simulink model "QDiff_ASGSM"  (R2024b)
settings: Solver=ode4  StartTime=0.0  StopTime=5  FixedStep=0.004  RelTol=1e-3
undefined symbols (not defined in the file or in its folder): DiscIntNeverNeededParam
libraries: aerolibutil x9, sharedutil x3, matrix_library x2, simulink_extras x1, simulink x1, sharedtransform x1
settings Model: Creator=danyy  LastModifiedBy=danyy

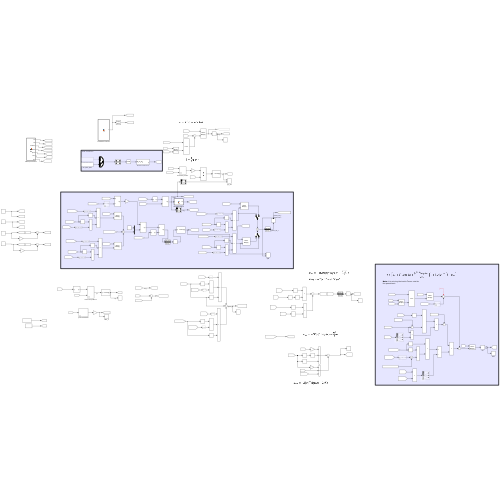
[thumbnail: Simulink's stored preview of the top-level diagram]
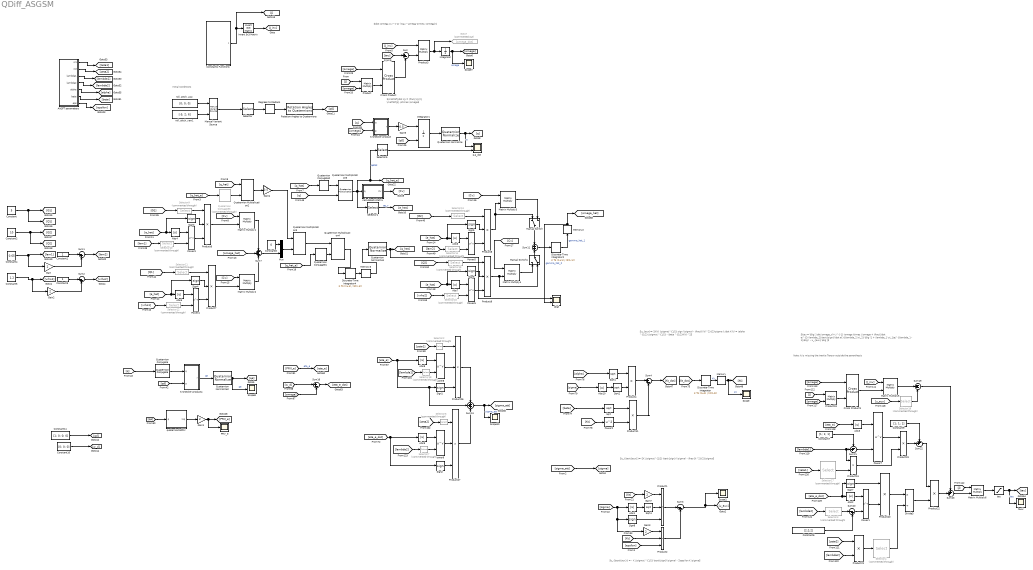
== system QDiff_ASGSM ==
  note: $u_{\text{aux}} = - K |\sigma| ^{1/2} \text{sign}(\sigma) - 2\epsilon K \sigma$
  note: $u_{\text{aux}}=-2K |\sigma|^{1/2} \text{sign} (\sigma) - \frac{K^2}{2}\sigma$
  note: $u_{aux}=-2K(t) |\sigma|^{1/2} sign (\sigma) - \frac{K(t)^2}{2}\sigma \\ \dot K(t) = \alpha ^{1/2} |\sigma| ^{1/2} - \beta ^{1/2}K(t)^2$
  note: $\tau = \Big [ \dot \omega_d + J^{-1} \omega \times J \omega + \frac{|\dot e|^{2-\lambda_2}\text{sign}(\dot e)}{\lambda_2 \xi_2} \Big (1 + \lambda_1 \xi_1|e|^{\lambda_1 - 1}\Big ) - u_{aux} \Big ]$
  note: Note: It is missing the Inertia Tensor outside
      | the parenthesis
  note: $\mathbf{\dot q} = \frac{1}{2} \mathbf{q} \otimes \omega$
  note: $\dot \omega = J^{-1} (\tau - \omega \times J \omega)$
  note: Initial Conditions
  ANSFT parameters : MATLAB Function  TreatAsAtomicUnit=on
  Abs{1..10} (10 alike) : Abs  SaturateOnIntegerOverflow=off
  Constant : Constant  Value=5
  Constant1 : Constant
  Constant10 : Constant  Value=[0; 0; 0]
  Constant11 : Constant  Value=[1; 0; 0; 0]
  Constant2 : Constant  Value=10
  Constant3 : Constant
  Constant4 : Constant  Value=0.65
  Constant5 : Constant  Value=1.2
  Constant6 : Constant  Value=[2;2;2]
  Constant7 : Constant  Value=[1; 1; 1]
  Constant8 : Constant  Value=0
  Constant9 : Constant  Value=[1; 1; 1]
  Constants Functions : MATLAB Function  TreatAsAtomicUnit=on
  Cross Product : matrix_library/Cross Product
  Cross Product1 : matrix_library/Cross Product
  Degrees to Radians : simulink_extras/Transformations/Degrees to Radians
  Discrete-Time Integrator : DiscreteIntegrator  IntegratorMethod=Integration: Trapezoidal  InitialCondition=[0; 0; 0]  SampleTime=0.004  ICPrevOutput=DiscIntNeverNeededParam  ICPrevScaledInput=DiscIntNeverNeededParam
  Discrete-Time Integrator2 : DiscreteIntegrator  IntegratorMethod=Integration: Trapezoidal  InitialCondition=[0; 0; 0]  SampleTime=0.004  ICPrevOutput=DiscIntNeverNeededParam  ICPrevScaledInput=DiscIntNeverNeededParam
  Discrete-Time Integrator4 : DiscreteIntegrator  IntegratorMethod=Integration: Trapezoidal  InitialCondition=[1; 0; 0; 0]  SampleTime=0.004  ICPrevOutput=DiscIntNeverNeededParam  ICPrevScaledInput=DiscIntNeverNeededParam
  Divide3 : Product  Inputs=*/
  Gain{,1..3,7} (5 alike) : Gain  Gain=2
  Gain4 : Gain  Gain=0.5
  Gain5 : Gain  Gain=0.5
  Goto7 : Goto  Commented=on  GotoTag=omega_dot
  Integrator : Integrator  InitialCondition=[0; 0; 0]
  Integrator1 : Integrator  InitialConditionSource=external
  Invert 3x3 Matrix : aerolibutil/Invert  3x3 Matrix
  Kronecker product : Subsystem
      mask Display: image('$imagefile'); % Use "Edit Image" on toolstrip to change.
  Kronecker product4 : Subsystem
  Manual Variant Source : simulink/Signal Routing/Manual Variant Source  NumChoices=2  LabelModeActiveChoice=V_2
  Manual Switch : ManualSwitch
  Manual Switch1 : ManualSwitch  CurrentSetting=0
  Matrix Multiply{1..6} (6 alike) : Product  Multiplication=Matrix(*)
  Memory : Memory  InitialCondition=[0; 0; 0]  InheritSampleTime=on
  Memory2 : Memory  InitialCondition=[0; 0; 0]  InheritSampleTime=on
  Memory3 : Memory  InitialCondition=[1; 0; 0; 0]  InheritSampleTime=on
  Mux : Mux  Inputs=2
  PRV_e : Scope
  Power{1,3..9} (8 alike) : Math  Operator=pow
  Power2 : Math  Operator=square
  Product : Product  Multiplication=Matrix(*)
  Product{1..2,6..9,26..27} (8 alike) : Product  Inputs=3
  Product{4,11,20..24} (7 alike) : Product
  Product19 : Product  Multiplication=Matrix(*)
  Product3 : Product  Multiplication=Matrix(*)
  Quaternion Conjugate : aerolibutil/Quaternion Conjugate
  Quaternion Conjugate1 : aerolibutil/Quaternion Conjugate
  Quaternion Conjugate2 : aerolibutil/Quaternion Conjugate
  Quaternion Conjugate3 : aerolibutil/Quaternion Conjugate  Commented=through
  Quaternion Multiplication{2..5} (4 alike) : aerolibutil/Quaternion Multiplication
  Quaternion Normalize : sharedutil/Quaternion Normalize  aMode=aMode
  Quaternion Normalize1 : sharedutil/Quaternion Normalize  aMode=aMode
  Quaternion Normalize2 : sharedutil/Quaternion Normalize  aMode=aMode
  Rotation Angles to Quaternions : sharedtransform/Rotation Angles to Quaternions  rotationOrder=ZYX  aMode=aMode
  Scope{,1,7..8,10} (5 alike) : Scope
  Selector : Selector  InputPortWidth=3  IndexOptions=Index vector (dialog)  Indices=[3 2 1]  OutputSizes=1
  Selector1 : Selector  InputPortWidth=4  IndexOptions=Index vector (dialog)  Indices=[2:4]  OutputSizes=1
  Selector{2..4,6..7,9..19} (16 alike) : Selector  Commented=through  InputPortWidth=6  IndexOptions=Index vector (dialog)  Indices=[4:6]  OutputSizes=1
  Selector5 : Selector  InputPortWidth=4  IndexOptions=Index vector (dialog)  Indices=[2:4]  OutputSizes=1
  Sign{1..8} (8 alike) : Signum
  Sqrt{,1..2,4} (4 alike) : Sqrt
  Sum : Sum  Inputs=|+-
  Sum1 : Sum  Inputs=|-+
  Sum11 : Sum  Inputs=+|+
  Sum16 : Sum  Inputs=|+-
  Sum19 : Sum  Inputs=-+-
  Sum2 : Sum  Inputs=|-+
  Sum20 : Sum  Inputs=|-+
  Sum21 : Sum  Inputs=-+|
  Sum22 : Sum  Inputs=++|
  Sum23 : Sum  Inputs=++|
  Sum24 : Sum  Inputs=+++
  Sum3 : Sum  Inputs=|--
  Sum4 : Sum  Inputs=|+-
  Sum7 : Sum  Inputs=+++
  calculateCvMatrix : MATLAB Function  TreatAsAtomicUnit=on
  q,q_dot : Scope  NumInputPorts=2
  qhat : Scope  NumInputPorts=2
  quaterniontoPRV : Subsystem
  "roll, pitch, yaw" : Constant  Value=[0; 0; 0]
  "roll, pitch, yaw1" : Constant  Value=[-3; 2; 6]
  tau : Saturate
  tauU : Scope
  wires:
  Memory3/1 -> Quaternion Normalize1/1
  [lam2] -> Selector14/1
  Sign6/1 -> Product9/2
  Selector10/1 -> Power3/2
  [G2] -> Selector13/1
  [q_hat_e] -> Quaternion Conjugate1/1
  Selector13/1 -> Product8/1
  Sign4/1 -> Product7/2
  Product6/1 -> Matrix Multiply1/2
  Selector15/1 -> Product9/1
  [Q1] -> Selector11/1
  Product7/1 -> Matrix Multiply2/2
  [Q2] -> Selector15/1
  [Cv] -> Matrix Multiply2/1
  Abs7/1 -> Power6/1
  [e_hat] -> Sign6/1, Abs7/1
  Quaternion Conjugate3/1 -> Quaternion Multiplication2/2
  Sign5/1 -> Product8/2
  Mux/1 -> Quaternion Multiplication3/2
  Matrix Multiply1/1 -> Sum7/1
  [q_hat] -> Quaternion Multiplication2/1
  Selector12/1 -> Power4/2
  Abs6/1 -> Power5/1
  Quaternion Conjugate1/1 -> Quaternion Multiplication4/2
  Power6/1 -> Product9/3
  Selector9/1 -> Product6/1
  Quaternion Multiplication2/1 -> Gain4/1
  [e_hat] -> Sign3/1, Abs4/1
  Power3/1 -> Product6/3
  Selector14/1 -> Power5/2
  Selector16/1 -> Power6/2
  Memory2/1 -> qhat/2, [omega_hat]  "gamma_hat_2"
  Constant8/1 -> Mux/1
  Quaternion Multiplication4/1 -> Discrete-Time Integrator4/1
  Abs5/1 -> Power4/1
  [Cv] -> Matrix Multiply1/1
  Gain4/1 -> Quaternion Multiplication3/1
  Sum7/1 -> Mux/2
  Power5/1 -> Product8/3
  [vrho2] -> Selector16/1
  Matrix Multiply2/1 -> Sum7/3
  [q_hat_e] -> Quaternion Conjugate3/1
  [e_hat] -> Sign5/1, Abs6/1
  Selector11/1 -> Product7/1
  Quaternion Normalize1/1 -> qhat/1, [q_hat]
  Discrete-Time Integrator2/1 -> Memory2/1  "gamma_hat_1"
  Product9/1 -> Manual Switch1/2, Matrix Multiply4/2
  [vrho1] -> Selector12/1
  [Cv] -> Matrix Multiply3/1
  Power4/1 -> Product7/3
  Matrix Multiply3/1 -> Manual Switch/2
  Matrix Multiply4/1 -> Manual Switch1/1
  Product8/1 -> Manual Switch/1, Matrix Multiply3/2
  [lam1] -> Selector10/1
  Discrete-Time Integrator4/1 -> Memory3/1
  [e_hat] -> Sign4/1, Abs5/1
  [G1] -> Selector9/1
  Abs4/1 -> Power3/1
  Sign3/1 -> Product6/2
  Quaternion Multiplication3/1 -> Quaternion Multiplication4/1
  Sum11/1 -> Discrete-Time Integrator2/1
  [omega_hat] -> Sum7/2
  [Cv] -> Matrix Multiply4/1
  Constant3/1 -> Sum2/1
  Constant/1 -> [G1], [Q1]
  Gain/1 -> Sum1/2
  Constant5/1 -> Gain2/1, [vrho1]
  Constant1/1 -> Sum1/1
  Gain2/1 -> Sum2/2
  Sum2/1 -> [vrho2]
  Constant4/1 -> Gain/1, [lam1]
  Constant2/1 -> [G2], [Q2]
  Sum1/1 -> [lam2]
  [q] -> Quaternion Multiplication5/2
  calculateCvMatrix/1(Cv) -> [Cv]
  [q_hat] -> Quaternion Conjugate2/1
  Quaternion Conjugate2/1 -> Quaternion Multiplication5/1
  Quaternion Multiplication5/1 -> Selector1/1, calculateCvMatrix/1(q), Selector5/1, [q_hat_e]  "qehat"
  Selector1/1 -> [e_hat]  "qe_v"
  Kronecker product4/1(r) -> Quaternion Normalize2/1  "qe"
  [qd] -> Kronecker product4/2(p)
  quaterniontoPRV/1(lnq) -> Gain1/1
  Quaternion Normalize2/1 -> Scope8/1, [qe]  "qe"
  Quaternion Conjugate/1 -> Kronecker product4/1(q)
  [q] -> Quaternion Conjugate/1
  [qe] -> quaterniontoPRV/1(q)
  Gain1/1 -> PRV_e/1, [PRV_e]
  [PRV_e] -> [eta_e]  "eta_e"
  [w_d] -> Sum16/1
  [omega] -> Sum16/2
  Sum16/1 -> [eta_e_dot]
  Product27/1 -> Sum24/3
  Selector18/1 -> Power8/2
  Selector6/1 -> Product27/1
  [eta_e] -> Sum24/2, Sign1/1, Abs8/1
  Selector7/1 -> Power9/2
  Abs8/1 -> Power8/1
  [eta_e_dot] -> Abs9/1, Sign2/1
  [lambda2] -> Selector7/1
  [lambda1] -> Selector18/1
  Product26/1 -> Sum24/1
  [zeta2] -> Selector6/1
  Abs9/1 -> Power9/1
  [zeta1] -> Selector2/1
  Sum24/1 -> Scope10/1, [sigma_att]  "sigma_att"
  Selector2/1 -> Product26/1
  Sign2/1 -> Product27/3
  Power9/1 -> Product27/2
  Sign1/1 -> Product26/3
  Power8/1 -> Product26/2
  Gain3/1 -> Product2/1
  Sum4/1 -> [Kt_dot]
  Sum3/1 -> Scope1/1, [u_aux]
  [Kt_dot] -> Discrete-Time Integrator/1
  [Kt] -> Power2/1
  [beta] -> Sqrt/1
  Product11/1 -> Sum4/2
  Product2/1 -> Sum3/2
  [Kt] -> Gain7/1
  [sigma_att] -> [sigma]
  Sign8/1 -> Product1/3
  Sqrt1/1 -> Product4/1
  [alpha] -> Sqrt1/1
  Power2/1 -> Product11/2
  Memory/1 -> Scope/1, [Kt]  "Kt"
  Gain7/1 -> Product1/1
  [sigma] -> Abs10/1
  [epsilon] -> Product2/3
  Product1/1 -> Sum3/1
  Abs10/1 -> Sqrt2/1
  Product4/1 -> Sum4/1
  Sqrt/1 -> Product11/1
  Sqrt2/1 -> Product4/2
  Discrete-Time Integrator/1 -> Memory/1  "Kt"
  [Kt] -> Product2/2
  Sqrt4/1 -> Product1/2
  [sigma] -> Abs1/1, Gain3/1, Sign8/1
  Abs1/1 -> Sqrt4/1
  Product23/1 -> Sum22/2
  Sum22/1 -> Product22/1
  Product20/1 -> Divide3/1
  ? -> Sum19/1
  Matrix Multiply5/1 -> Sum19/2
  Matrix Multiply6/1 -> tau/1
  [lambda2] -> Selector3/1
  Product21/1 -> Selector4/1
  Sum21/1 -> Power7/2
  [lambda1] -> Product24/1, Sum21/2
  Constant9/1 -> Sum22/1
  [J_inv] -> Matrix Multiply5/1
  [J] -> Product19/1
  [u_aux] -> Selector19/1
  Product19/1 -> Cross Product1/2
  [lambda2] -> Product21/2
  tau/1 -> tauU/1, [tau]  "tau"
  Sum23/1 -> Matrix Multiply6/2
  Constant6/1 -> Sum20/2
  [eta_e_dot] -> Sign7/1, Abs2/1
  Cross Product1/1 -> Matrix Multiply5/2
  Selector19/1 -> Sum19/3
  Selector4/1 -> Divide3/2
  [eta_e] -> Abs3/1
  Sum19/1 -> Sum23/1
  [omega] -> Product19/2
  [zeta2] -> Product21/1
  Abs2/1 -> Power1/1
  Constant7/1 -> Sum21/1
  Power7/1 -> Product23/1
  Selector17/1 -> Product24/2
  [J] -> Matrix Multiply6/1
  [omega] -> Cross Product1/1
  Sum20/1 -> Power1/2
  Sign7/1 -> Product20/1
  Product22/1 -> Sum23/2
  [zeta1] -> Selector17/1
  Product24/1 -> Product23/2
  Selector3/1 -> Sum20/1
  Divide3/1 -> Product22/2
  Power1/1 -> Product20/2
  Abs3/1 -> Power7/1
  Product3/1 -> Goto7/1, Integrator/1
  [q] -> Kronecker product/1(q)
  [omega] -> Cross Product/1
  Sum/1 -> Product3/2
  [omega] -> Kronecker product/2(p)
  [omega] -> Product/2
  Quaternion Normalize/1 -> q,q_dot/1, [q]  "q"
  Product/1 -> Cross Product/2
  Integrator1/1 -> Quaternion Normalize/1
  Cross Product/1 -> Sum/2
  Integrator/1 -> Scope7/1, [omega]  "omega"
  [tau] -> Sum/1
  [q0] -> Integrator1/2
  [J_inv] -> Product3/1
  Gain5/1 -> Integrator1/1
  Kronecker product/1(r) -> Gain5/1
  [J] -> Product/1
  Selector/1 -> Degrees to Radians/1
  Rotation Angles to Quaternions/1 -> [q0]
  "roll, pitch, yaw1"/1 -> Manual Variant Source/2
  "roll, pitch, yaw"/1 -> Manual Variant Source/1
  Manual Variant Source/1 -> Selector/1
  Degrees to Radians/1 -> Rotation Angles to Quaternions/1
  Constants Functions/1(J) -> [J], Invert 3x3 Matrix/1
  Invert 3x3 Matrix/1 -> [J_inv]
  ANSFT parameters/2(xi2) -> [zeta2]
  ANSFT parameters/6(beta) -> [beta]
  ANSFT parameters/1(xi1) -> [zeta1]
  ANSFT parameters/5(alpha) -> [alpha]
  ANSFT parameters/4(lambda2) -> [lambda2]
  ANSFT parameters/3(lambda1) -> [lambda1]
  Constant10/1 -> [w_d]
  Constant11/1 -> [qd]
  ANSFT parameters/7(eps) -> [epsilon]
  Manual Switch/1 -> Sum11/1
  Manual Switch1/1 -> Sum11/2
  Selector5/1 -> q,q_dot/2

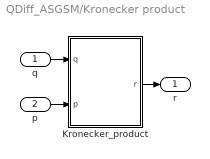
== system QDiff_ASGSM/Kronecker product ==
  q : Inport
  p : Inport  Port=2
  Kronecker_product : MATLAB Function  TreatAsAtomicUnit=on
  r : Outport
  wires:
  q/1 -> Kronecker_product/1(q)
  p/1 -> Kronecker_product/2(p)
  Kronecker_product/1(r) -> r/1

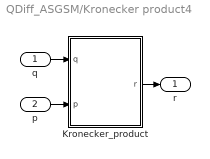
== system QDiff_ASGSM/Kronecker product4 ==
  q : Inport
  p : Inport  Port=2
  Kronecker_product : MATLAB Function  TreatAsAtomicUnit=on
  r : Outport
  wires:
  q/1 -> Kronecker_product/1(q)
  p/1 -> Kronecker_product/2(p)
  Kronecker_product/1(r) -> r/1

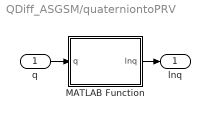
== system QDiff_ASGSM/quaterniontoPRV ==
  q : Inport
  MATLAB Function : MATLAB Function  TreatAsAtomicUnit=on
  lnq : Outport
  wires:
  MATLAB Function/1(lnq) -> lnq/1
  q/1 -> MATLAB Function/1(q)

== matlab function QDiff_ASGSM/Kronecker product/Kronecker_product ==
  data: q input; r output size=[4 1]; p input
function r = fcn(q, p)

%{
    Function to describe in matrix math the Kronecker product between
    two quaternions
    
    r = p kronecker q
    %}

    len = length(p);

    if len == 3 && length(q) == 4
        p1 = [0; p];
        q0 = q(1);
        q1 = q(2);
        q2 = q(3);
        q3 = q(4);
        
        % skew symmetric matrix
        q_matrix = [q0, -q1, -q2, -q3;
                  q1, q0, -q3, q2;
                  q2, q3, q0, -q1;
                  q3, -q2, q1, q0];
        
        r = q_matrix * p1;

    elseif len == 4
        q0 = q(1);
        q1 = q(2);
        q2 = q(3);
        q3 = q(4);
        
        % skew symmetric matrix
        q_matrix = [q0, -q1, -q2, -q3;
                  q1, q0, -q3, q2;
                  q2, q3, q0, -q1;
                  q3, -q2, q1, q0];
        
        r = q_matrix * p;

    else
        error('Quaternions dimensions do not match')
    end

== matlab function QDiff_ASGSM/Constants Functions ==
  data: J output
function J  = fcn



% Jxx =  0.0411; % kg m²
% Jyy = 0.0478; % kg m²
% Jzz = 0.0599; % kg m²

Jxx = 0.028;
Jyy = 0.031;
Jzz = 0.048;

J = [Jxx, 0, 0;
     0, Jyy, 0;
     0, 0, Jzz];

== matlab function QDiff_ASGSM/calculateCvMatrix ==
  data: q input; Cv output
function Cv = fcn(q)

q0 = q(1);
q1 = q(2);
q2 = q(3);
q3 = q(4);

Cv = [q0, -q3, q2;
      q3, q0, -q1;
      -q2, q1, q0] * 0.5;

Cv = pinv(Cv);

== matlab function QDiff_ASGSM/quaterniontoPRV/MATLAB Function ==
  data: q input; lnq output size=[3 1]
function lnq = fcn(q)

if length(q) == 4
    q0 = q(1);
    q_vec = [q(2); q(3); q(4)];

    if norm(q_vec) == 0
        lnq = [0; 0; 0];
    else
        % q0 = real(q0);
        lnq = (q_vec / (norm(q_vec)) ) * acos(q0);
    end
else
    error('Input must be a vector 4 by 1 (Quaternion)')
end

== matlab function QDiff_ASGSM/Kronecker product4/Kronecker_product ==
  data: q input; r output size=[4 1]; p input
function r = fcn(q, p)

%{
    Function to describe in matrix math the Kronecker product between
    two quaternions
    
    r = p kronecker q
    %}

    len = length(p);

    if len == 3 && length(q) == 4
        p1 = [0; p];
        q0 = q(1);
        q1 = q(2);
        q2 = q(3);
        q3 = q(4);
        
        % skew symmetric matrix
        q_matrix = [q0, -q1, -q2, -q3;
                  q1, q0, -q3, q2;
                  q2, q3, q0, -q1;
                  q3, -q2, q1, q0];
        
        r = q_matrix * p1;

    elseif len == 4
        q0 = q(1);
        q1 = q(2);
        q2 = q(3);
        q3 = q(4);
        
        % skew symmetric matrix
        q_matrix = [q0, -q1, -q2, -q3;
                  q1, q0, -q3, q2;
                  q2, q3, q0, -q1;
                  q3, -q2, q1, q0];
        
        r = q_matrix * p;

    else
        error('Quaternions dimensions do not match')
    end

== matlab function QDiff_ASGSM/ANSFT parameters ==
  data: xi1 output; xi2 output; lambda1 output; lambda2 output; alpha output; beta output; eps output
function [xi1, xi2, lambda1, lambda2, alpha, beta, eps] = fcn

%% Constantes de la Superficie deslizante
% zeta1 parecido a una ganancia proporcional
xi1 = [1; 1; 1];
%zeta2 parecido a una ganancia derivatida
xi2 = [2; 2; 2];
% lambda 1 > lambda2
lambda1 = [2; 2; 2];
% 1 < lambda2 < 2
lambda2 = [1.33; 1.33; 1.33];
%% Constantes del control auxiliar
%minimize sigma
alpha = [2.5; 2.5; 1.25];
%aumetnar control, aumentar energía del sistema
beta = [0.05; 0.05; 0.25];

eps = [0.2; 0.2; 0.2];
